simulink subsystem "IMU2"  (R2021a)
settings: Solver=VariableStepAuto  StartTime=0.0  StopTime=10.0  RelTol=1e-3
undefined symbols (not defined in the file): imu1, imu2, Ts
libraries: simulink x8, dspsrcs4 x3, dspmtrx3 x2
settings Model: Creator=Laura  LastModifiedBy=Laura

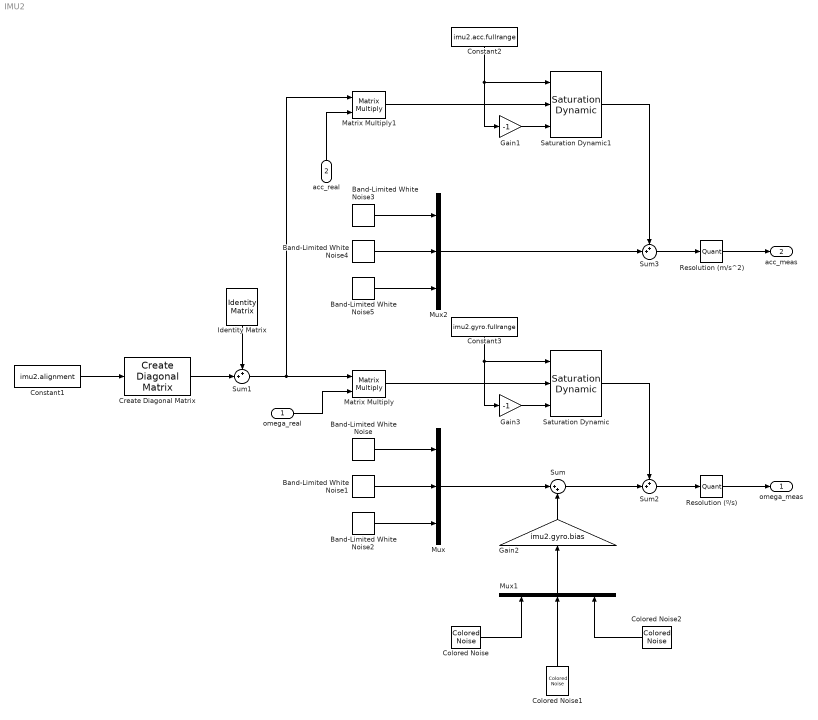
== system IMU2 ==
  omega_real : Inport
  acc_real : Inport  Port=2
  Band-Limited White Noise : simulink/Sources/Band-Limited White Noise  Cov=imu2.gyro.noisepower(1)  Ts=Ts  seed=[23341]
  Band-Limited White Noise1 : simulink/Sources/Band-Limited White Noise  Cov=imu2.gyro.noisepower(2)  Ts=Ts  seed=[23341]
  Band-Limited White Noise2 : simulink/Sources/Band-Limited White Noise  Cov=imu2.gyro.noisepower(3)  Ts=Ts  seed=[23341]
  Band-Limited White Noise3 : simulink/Sources/Band-Limited White Noise  Cov=imu1.acc.noisepower(1)  Ts=Ts  seed=[23341]
  Band-Limited White Noise4 : simulink/Sources/Band-Limited White Noise  Cov=imu1.acc.noisepower(2)  Ts=Ts  seed=[23341]
  Band-Limited White Noise5 : simulink/Sources/Band-Limited White Noise  Cov=imu1.acc.noisepower(3)  Ts=Ts  seed=[23341]
  Colored Noise : dspsrcs4/Colored Noise  Color=pink  InverseFrequencyPower=1  BoundedOutput=off  NumChannels=1  OutputDataType=double  SamplesPerFrame=1  SampleTime=Ts  RandomStream=mt19937ar with seed  Seed=67  SimulateUsing=Interpreted execution
      settings: SourceProductBaseCode=DS
  Colored Noise1 : dspsrcs4/Colored Noise  Color=pink  InverseFrequencyPower=1  BoundedOutput=off  NumChannels=1  OutputDataType=double  SamplesPerFrame=1  SampleTime=Ts  RandomStream=mt19937ar with seed  Seed=67  SimulateUsing=Interpreted execution
      settings: SourceProductBaseCode=DS
  Colored Noise2 : dspsrcs4/Colored Noise  Color=pink  InverseFrequencyPower=1  BoundedOutput=off  NumChannels=1  OutputDataType=double  SamplesPerFrame=1  SampleTime=Ts  RandomStream=mt19937ar with seed  Seed=67  SimulateUsing=Interpreted execution
      settings: SourceProductBaseCode=DS
  Constant1 : Constant  Value=imu2.alignment
  Constant2 : Constant  Value=imu2.acc.fullrange
  Constant3 : Constant  Value=imu2.gyro.fullrange
  Create Diagonal Matrix : dspmtrx3/Create Diagonal Matrix
      settings: SourceProductBaseCode=DS
  Gain1 : Gain  Gain=-1
  Gain2 : Gain  Gain=imu2.gyro.bias
  Gain3 : Gain  Gain=-1
  Identity Matrix : dspmtrx3/Identity Matrix  Inherit=off  N=3  Ts=1  dataType=double  isSigned=on  wordLen=16  udDataType=sfix(16)  fracBitsMode=Best precision  numFracBits=15  OutDataTypeStr=double  LastOutDataTypeStr=double
  Matrix Multiply : Product  Multiplication=Matrix(*)
  Matrix Multiply1 : Product  Multiplication=Matrix(*)
  Mux : Mux  Inputs=3
  Mux1 : Mux  Inputs=3
  Mux2 : Mux  Inputs=3
  Resolution (m/s^2) : Quantizer  QuantizationInterval=imu2.acc.quantization  LinearizeAsGain=off
  Resolution (º/s) : Quantizer  QuantizationInterval=imu2.gyro.quantization  LinearizeAsGain=off
  Saturation Dynamic : simulink/Discontinuities/Saturation Dynamic  OutMin=[]  OutMax=[]  OutDataTypeStr=Inherit: Same as second input  OutDataType=fixdt(1, 16)  OutScaling=2^-10  DoSatur=off
  Saturation Dynamic1 : simulink/Discontinuities/Saturation Dynamic  OutMin=[]  OutMax=[]  OutDataTypeStr=Inherit: Same as second input  OutDataType=fixdt(1, 16)  OutScaling=2^-10  DoSatur=off
  Sum : Sum  Inputs=|++
  Sum1 : Sum  Inputs=++|
  Sum2 : Sum  Inputs=++|
  Sum3 : Sum  Inputs=++|
  omega_meas : Outport
  acc_meas : Outport  Port=2
  wires:
  Band-Limited White Noise2/1 -> Mux/3
  Band-Limited White Noise1/1 -> Mux/2
  Band-Limited White Noise/1 -> Mux/1
  Mux/1 -> Sum/1
  Saturation Dynamic/1 -> Sum2/1
  Sum/1 -> Sum2/2
  Constant3/1 -> Gain3/1, Saturation Dynamic/1
  Gain3/1 -> Saturation Dynamic/3
  Identity Matrix/1 -> Sum1/1
  Sum1/1 -> Matrix Multiply1/1, Matrix Multiply/1
  omega_real/1 -> Matrix Multiply/2
  Matrix Multiply/1 -> Saturation Dynamic/2
  Sum2/1 -> Resolution (º/s)/1
  Colored Noise1/1 -> Mux1/2
  Gain2/1 -> Sum/2
  Colored Noise/1 -> Mux1/1
  Colored Noise2/1 -> Mux1/3
  Mux1/1 -> Gain2/1
  Constant1/1 -> Create Diagonal Matrix/1
  Create Diagonal Matrix/1 -> Sum1/2
  Resolution (º/s)/1 -> omega_meas/1
  Band-Limited White Noise3/1 -> Mux2/1
  Mux2/1 -> Sum3/2
  Band-Limited White Noise5/1 -> Mux2/3
  Band-Limited White Noise4/1 -> Mux2/2
  Resolution (m/s^2)/1 -> acc_meas/1
  Sum3/1 -> Resolution (m/s^2)/1
  Matrix Multiply1/1 -> Saturation Dynamic1/2
  Gain1/1 -> Saturation Dynamic1/3
  Constant2/1 -> Saturation Dynamic1/1, Gain1/1
  Saturation Dynamic1/1 -> Sum3/1
  acc_real/1 -> Matrix Multiply1/2
